simulink model "Speed_Bump"  (R2023b)
settings: Solver=VariableStepAuto  StartTime=0.0  StopTime=10  RelTol=1e-3
values from neighbouring files (symbols this model uses):
  a = 1.35    [Parameters.m]
  b = 1.5    [Parameters.m]
  d = 3    [Parameters.m]
  g = 9.81    [Parameters.m]
  I = 650    [Parameters.m]
  Kt = 14e4    (= 140000)    [Parameters.m]
  L = 3.7    [Parameters.m]
  Mw = 20    [Parameters.m]
  v = [1, 2, 3, 5, 8, 10]    [Parameters.m]
libraries: CarModelLibrary x6, SpeedBumpLibrary x4, simulink x4
settings Model: Creator=arturogonzalez  LastModifiedBy=franc
settings SolverCC: AlgebraicLoopSolver=TrustRegion
settings DebuggingCC: UnconnectedInputMsg=warning  UnconnectedOutputMsg=warning  UnconnectedLineMsg=warning
settings ModelReferenceCC: EnableRefExpFcnMdlSchedulingChecks=on

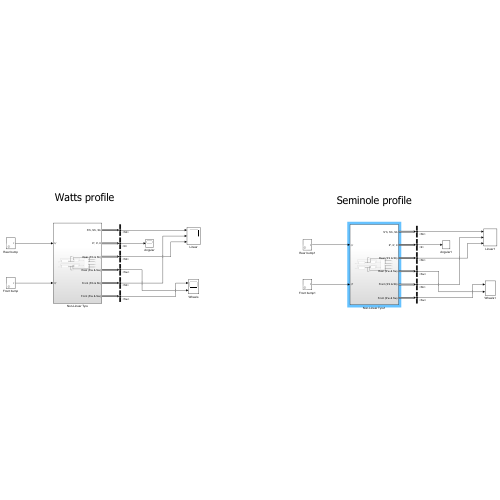
[thumbnail: Simulink's stored preview of the top-level diagram]
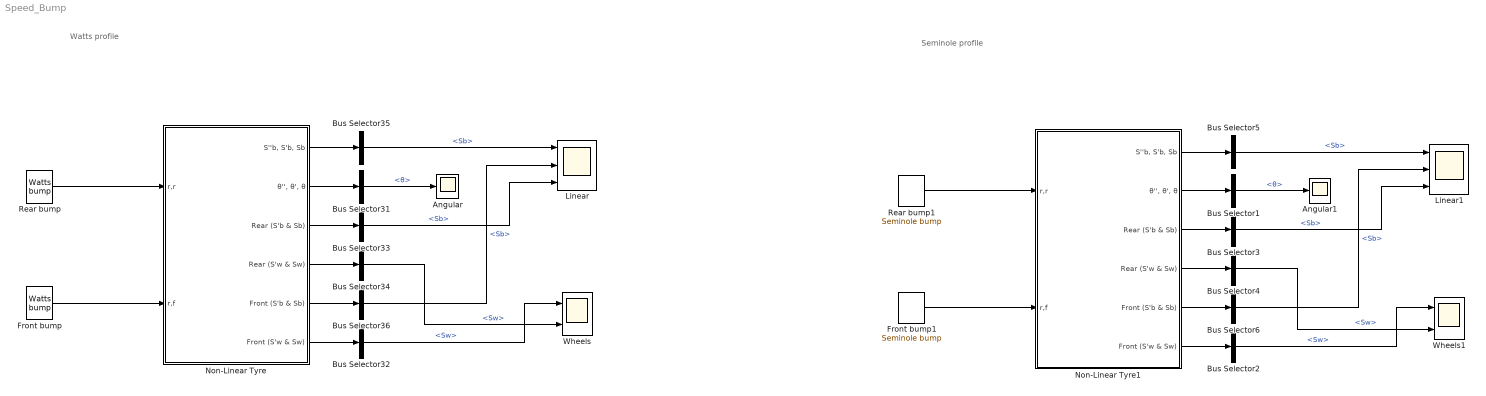
== system Speed_Bump ==
  note: Watts profile
  note: Seminole profile
  Angular : Scope
  Angular1 : Scope
  Bus Selector1 : BusSelector  OutputSignals=θ
  Bus Selector{2,4,32,34} (4 alike) : BusSelector  OutputSignals=Sw
  Bus Selector{3,5..6,33,35..36} (6 alike) : BusSelector  OutputSignals=Sb
  Bus Selector31 : BusSelector  OutputSignals=θ
  Front bump : SpeedBumpLibrary/Watts bump  h=h  L=L  v=v(5)  delta=0  n=12
  Front bump1 : SpeedBumpLibrary/Seminole bump  h=h  d=d  L=L+d  v=v(5)  delta=0  n=5
  Linear : Scope  NumInputPorts=3
  Linear1 : Scope  NumInputPorts=3
  Non-Linear Tyre : Subsystem
  Non-Linear Tyre1 : Subsystem
  Rear bump : SpeedBumpLibrary/Watts bump  h=h  L=L  v=v(5)  delta=a+b  n=12
  Rear bump1 : SpeedBumpLibrary/Seminole bump  h=h  d=d  L=L+d  v=v(5)  delta=a+b  n=5
  Wheels : Scope  NumInputPorts=2
  Wheels1 : Scope  NumInputPorts=2
  wires:
  Non-Linear Tyre/2("θ'', θ', θ") -> Bus Selector31/1
  Non-Linear Tyre/6(Front (S'w & Sw)) -> Bus Selector32/1
  Bus Selector35/1 -> Linear/1  "<Sb>"
  Non-Linear Tyre/4(Rear (S'w & Sw)) -> Bus Selector34/1
  Non-Linear Tyre/5(Front (S'b & Sb)) -> Bus Selector36/1
  Non-Linear Tyre/1("S''b, S'b, Sb") -> Bus Selector35/1
  Non-Linear Tyre/3(Rear (S'b & Sb)) -> Bus Selector33/1
  Front bump/1 -> Non-Linear Tyre/2(r,f)
  Rear bump/1 -> Non-Linear Tyre/1(r,r)
  Bus Selector31/1 -> Angular/1  "<θ>"
  Bus Selector33/1 -> Linear/3  "<Sb>"
  Bus Selector36/1 -> Linear/2  "<Sb>"
  Bus Selector34/1 -> Wheels/2  "<Sw>"
  Bus Selector32/1 -> Wheels/1  "<Sw>"
  Bus Selector1/1 -> Angular1/1  "<θ>"
  Bus Selector6/1 -> Linear1/2  "<Sb>"
  Bus Selector4/1 -> Wheels1/2  "<Sw>"
  Non-Linear Tyre1/3(Rear (S'b & Sb)) -> Bus Selector3/1
  Bus Selector3/1 -> Linear1/3  "<Sb>"
  Bus Selector2/1 -> Wheels1/1  "<Sw>"
  Non-Linear Tyre1/5(Front (S'b & Sb)) -> Bus Selector6/1
  Non-Linear Tyre1/6(Front (S'w & Sw)) -> Bus Selector2/1
  Non-Linear Tyre1/1("S''b, S'b, Sb") -> Bus Selector5/1
  Rear bump1/1 -> Non-Linear Tyre1/1(r,r)
  Bus Selector5/1 -> Linear1/1  "<Sb>"
  Non-Linear Tyre1/2("θ'', θ', θ") -> Bus Selector1/1
  Front bump1/1 -> Non-Linear Tyre1/2(r,f)
  Non-Linear Tyre1/4(Rear (S'w & Sw)) -> Bus Selector4/1

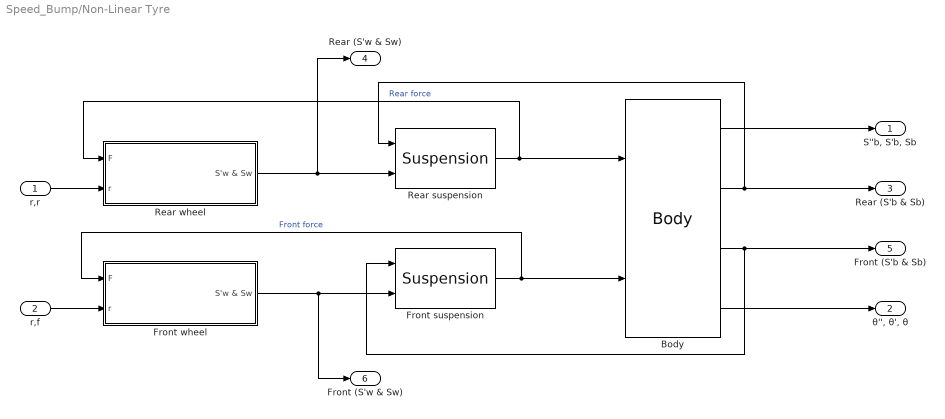
== system Speed_Bump/Non-Linear Tyre ==
  r,r : Inport
  r,f : Inport  Port=2
  Body : CarModelLibrary/Body  mb=Mb  I=I  a=a  b=b
  Front suspension : CarModelLibrary/Suspension  ks=Ks  ksstiff=Kstiff  x0=x0  csb=Csc  csr=Cse
  Front wheel : Subsystem  AncestorBlock=CarModelLibrary/Wheel  mask{mw=Mw, Kt=Kt, g=g}
      mask prompts: mw "Wheel Mass (Kg)"; Kt "Tyre Stiffness"; g "Gravitational acceleration"
  Rear suspension : CarModelLibrary/Suspension  ks=Ks  ksstiff=Kstiff  x0=x0  csb=Csc  csr=Cse
  Rear wheel : Subsystem  AncestorBlock=CarModelLibrary/Wheel  mask{mw=Mw, Kt=Kt, g=g}
      mask prompts: mw "Wheel Mass (Kg)"; Kt "Tyre Stiffness"; g "Gravitational acceleration"
  "S''b, S'b, Sb" : Outport
  "θ'', θ', θ" : Outport  Port=2
  Rear (S'b & Sb) : Outport  Port=3
  Rear (S'w & Sw) : Outport  Port=4
  Front (S'b & Sb) : Outport  Port=5
  Front (S'w & Sw) : Outport  Port=6
  wires:
  Body/1 -> "S''b, S'b, Sb"/1
  Body/2 -> Rear suspension/1, Rear (S'b & Sb)/1
  Front wheel/1(S'w & Sw) -> Front suspension/2, Front (S'w & Sw)/1
  Rear wheel/1(S'w & Sw) -> Rear suspension/2, Rear (S'w & Sw)/1
  Body/4 -> "θ'', θ', θ"/1
  Body/3 -> Front suspension/1, Front (S'b & Sb)/1
  Rear suspension/1 -> Body/1, Rear wheel/1(F)  "Rear force"
  r,r/1 -> Rear wheel/2(r)
  r,f/1 -> Front wheel/2(r)
  Front suspension/1 -> Front wheel/1(F), Body/2  "Front force"

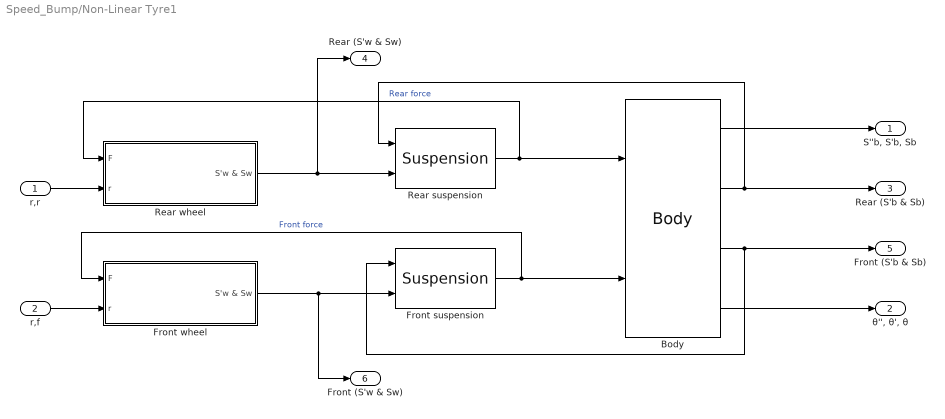
== system Speed_Bump/Non-Linear Tyre1 ==
  r,r : Inport
  r,f : Inport  Port=2
  Body : CarModelLibrary/Body  mb=Mb  I=I  a=a  b=b
  Front suspension : CarModelLibrary/Suspension  ks=Ks  ksstiff=Kstiff  x0=x0  csb=Csc  csr=Cse
  Front wheel : Subsystem  AncestorBlock=CarModelLibrary/Wheel  mask{mw=Mw, Kt=Kt, g=g}
      mask prompts: mw "Wheel Mass (Kg)"; Kt "Tyre Stiffness"; g "Gravitational acceleration"
  Rear suspension : CarModelLibrary/Suspension  ks=Ks  ksstiff=Kstiff  x0=x0  csb=Csc  csr=Cse
  Rear wheel : Subsystem  AncestorBlock=CarModelLibrary/Wheel  mask{mw=Mw, Kt=Kt, g=g}
      mask prompts: mw "Wheel Mass (Kg)"; Kt "Tyre Stiffness"; g "Gravitational acceleration"
  "S''b, S'b, Sb" : Outport
  "θ'', θ', θ" : Outport  Port=2
  Rear (S'b & Sb) : Outport  Port=3
  Rear (S'w & Sw) : Outport  Port=4
  Front (S'b & Sb) : Outport  Port=5
  Front (S'w & Sw) : Outport  Port=6
  wires:
  Body/1 -> "S''b, S'b, Sb"/1
  Body/2 -> Rear suspension/1, Rear (S'b & Sb)/1
  Front wheel/1(S'w & Sw) -> Front suspension/2, Front (S'w & Sw)/1
  Rear wheel/1(S'w & Sw) -> Rear suspension/2, Rear (S'w & Sw)/1
  Body/4 -> "θ'', θ', θ"/1
  Body/3 -> Front suspension/1, Front (S'b & Sb)/1
  Rear suspension/1 -> Body/1, Rear wheel/1(F)  "Rear force"
  r,r/1 -> Rear wheel/2(r)
  r,f/1 -> Front wheel/2(r)
  Front suspension/1 -> Front wheel/1(F), Body/2  "Front force"

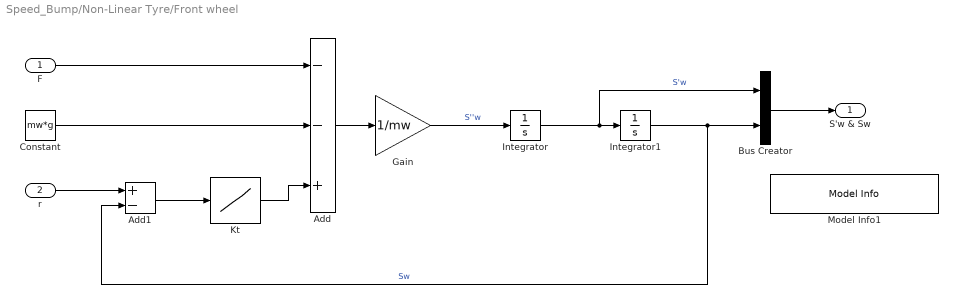
== system Speed_Bump/Non-Linear Tyre/Front wheel ==
  F : Inport
  r : Inport  Port=2
  Add : Sum  Inputs=--+
  Add1 : Sum  Inputs=+-
  Bus Creator : BusCreator  Inputs=2
  Constant : Constant  Value=mw*g
  Gain : Gain  Gain=1/mw
  Integrator : Integrator
  Integrator1 : Integrator
  Kt : Lookup_n-D  NumberOfTableDimensions=1  BreakpointsForDimension1=[-1, 0, 1]  Table=[0, 0, Kt]  InternalRulePriority=Speed  RndMeth=Simplest
  Model Info1 : simulink/Model-Wide Utilities/Model Info  Frame=on  DisplayStringWithTags=m * S''w = -F + Kt (r-S) - m*g  HorizontalTextAlignment=Center  LeftAlignmentValue=0.5
  S'w & Sw : Outport
  wires:
  Kt/1 -> Add/3
  F/1 -> Add/1
  Constant/1 -> Add/2
  Gain/1 -> Integrator/1  "S''w"
  Add/1 -> Gain/1
  Integrator1/1 -> Add1/2, Bus Creator/2  "Sw"
  Bus Creator/1 -> S'w & Sw/1
  Integrator/1 -> Integrator1/1, Bus Creator/1  "S'w"
  Add1/1 -> Kt/1
  r/1 -> Add1/1

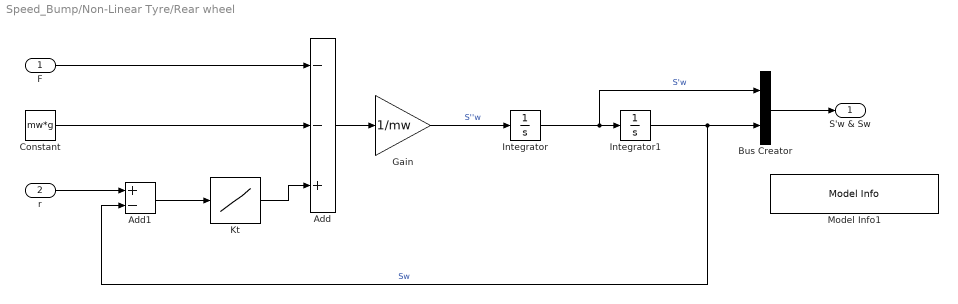
== system Speed_Bump/Non-Linear Tyre/Rear wheel ==
  F : Inport
  r : Inport  Port=2
  Add : Sum  Inputs=--+
  Add1 : Sum  Inputs=+-
  Bus Creator : BusCreator  Inputs=2
  Constant : Constant  Value=mw*g
  Gain : Gain  Gain=1/mw
  Integrator : Integrator
  Integrator1 : Integrator
  Kt : Lookup_n-D  NumberOfTableDimensions=1  BreakpointsForDimension1=[-1, 0, 1]  Table=[0, 0, Kt]  InternalRulePriority=Speed  RndMeth=Simplest
  Model Info1 : simulink/Model-Wide Utilities/Model Info  Frame=on  DisplayStringWithTags=m * S''w = -F + Kt (r-S) - m*g  HorizontalTextAlignment=Center  LeftAlignmentValue=0.5
  S'w & Sw : Outport
  wires:
  Kt/1 -> Add/3
  F/1 -> Add/1
  Constant/1 -> Add/2
  Gain/1 -> Integrator/1  "S''w"
  Add/1 -> Gain/1
  Integrator1/1 -> Add1/2, Bus Creator/2  "Sw"
  Bus Creator/1 -> S'w & Sw/1
  Integrator/1 -> Integrator1/1, Bus Creator/1  "S'w"
  Add1/1 -> Kt/1
  r/1 -> Add1/1

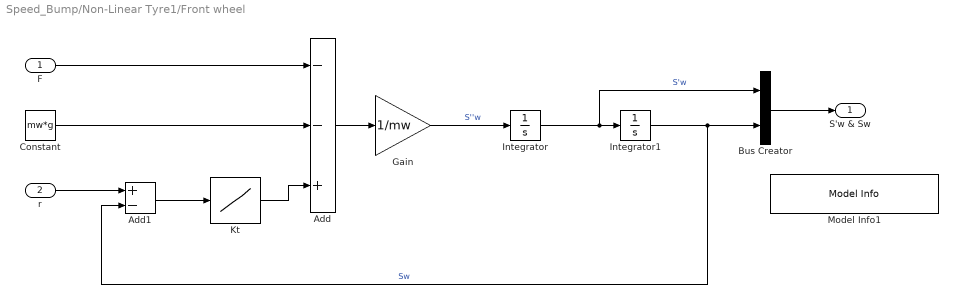
== system Speed_Bump/Non-Linear Tyre1/Front wheel ==
  F : Inport
  r : Inport  Port=2
  Add : Sum  Inputs=--+
  Add1 : Sum  Inputs=+-
  Bus Creator : BusCreator  Inputs=2
  Constant : Constant  Value=mw*g
  Gain : Gain  Gain=1/mw
  Integrator : Integrator
  Integrator1 : Integrator
  Kt : Lookup_n-D  NumberOfTableDimensions=1  BreakpointsForDimension1=[-1, 0, 1]  Table=[0, 0, Kt]  InternalRulePriority=Speed  RndMeth=Simplest
  Model Info1 : simulink/Model-Wide Utilities/Model Info  Frame=on  DisplayStringWithTags=m * S''w = -F + Kt (r-S) - m*g  HorizontalTextAlignment=Center  LeftAlignmentValue=0.5
  S'w & Sw : Outport
  wires:
  Kt/1 -> Add/3
  F/1 -> Add/1
  Constant/1 -> Add/2
  Gain/1 -> Integrator/1  "S''w"
  Add/1 -> Gain/1
  Integrator1/1 -> Add1/2, Bus Creator/2  "Sw"
  Bus Creator/1 -> S'w & Sw/1
  Integrator/1 -> Integrator1/1, Bus Creator/1  "S'w"
  Add1/1 -> Kt/1
  r/1 -> Add1/1

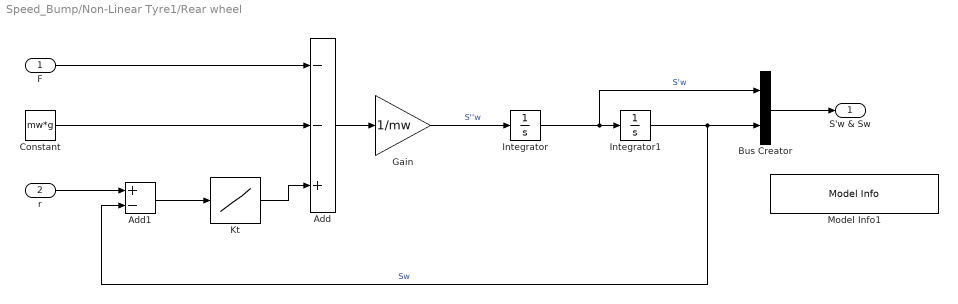
== system Speed_Bump/Non-Linear Tyre1/Rear wheel ==
  F : Inport
  r : Inport  Port=2
  Add : Sum  Inputs=--+
  Add1 : Sum  Inputs=+-
  Bus Creator : BusCreator  Inputs=2
  Constant : Constant  Value=mw*g
  Gain : Gain  Gain=1/mw
  Integrator : Integrator
  Integrator1 : Integrator
  Kt : Lookup_n-D  NumberOfTableDimensions=1  BreakpointsForDimension1=[-1, 0, 1]  Table=[0, 0, Kt]  InternalRulePriority=Speed  RndMeth=Simplest
  Model Info1 : simulink/Model-Wide Utilities/Model Info  Frame=on  DisplayStringWithTags=m * S''w = -F + Kt (r-S) - m*g  HorizontalTextAlignment=Center  LeftAlignmentValue=0.5
  S'w & Sw : Outport
  wires:
  Kt/1 -> Add/3
  F/1 -> Add/1
  Constant/1 -> Add/2
  Gain/1 -> Integrator/1  "S''w"
  Add/1 -> Gain/1
  Integrator1/1 -> Add1/2, Bus Creator/2  "Sw"
  Bus Creator/1 -> S'w & Sw/1
  Integrator/1 -> Integrator1/1, Bus Creator/1  "S'w"
  Add1/1 -> Kt/1
  r/1 -> Add1/1
